simulink model "quadcopter_model"  (R2026a)
settings: Solver=VariableStepAuto  StopTime=60
undefined symbols (not defined in the file): g, Ixx, Iyy, Izz, m
libraries: mpclib x1, uavutilslib x1
settings Model: Creator=Krrrrish  LastModifiedBy=Krrrrish

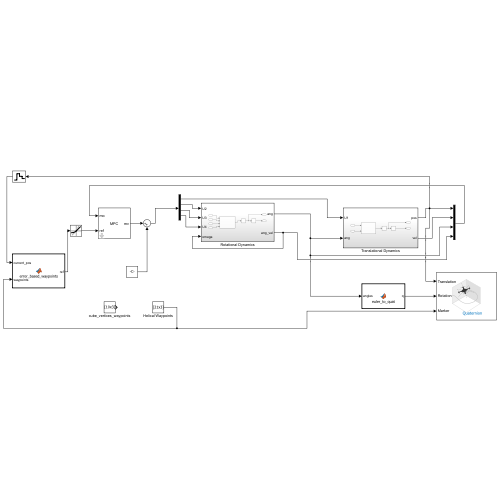
[thumbnail: Simulink's stored preview of the top-level diagram]
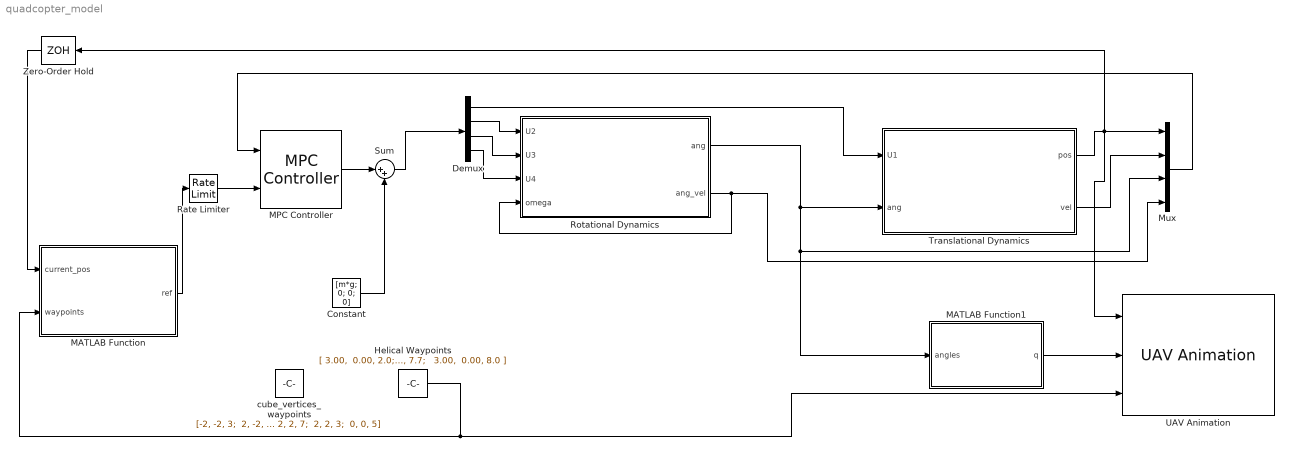
== system quadcopter_model ==
  Constant : Constant  Value=[m*g; 0; 0; 0]
  Demux : Demux
  Helical Waypoints : Constant  Value=|
      | [ 3.00,  0.00, 2.0;
      |   2.43,  1.76, 2.3;
      |   0.93,  2.85, 2.6;
      |  -0.93,  2.85, 2.9;
      |  -2.43,  1.76, 3.2;
      |  -3.00,  0.00, 3.5;
      |  -2.43, -1.76, 3.8;
      |  -0.93, -2.85, 4.1;
      |   0.93, -2.85, 4.4;
      |   2.43, -1.76, 4.7;
      |   3.00,  0.00, 5.0;
      |   2.43,  1.76, 5.3;
      |   0.93,  2.85, 5.6;
      |  -0.93,  2.85, 5.9;
      |  -2.43,  1.76, 6.2;
      |  -3.00,  0.00, 6.5;
      |  -2.43, -1.76, 6.8;
      |  -0.93, -2.85, 7.1;
      |   0.93, -2.85, 7.4;
      |   2.43, -1.76, 7.7;
      |   3.00,  0.00, 8.0 ]
  MATLAB Function : MATLAB Function  TreatAsAtomicUnit=on
  MATLAB Function1 : MATLAB Function  TreatAsAtomicUnit=on
  MPC Controller : mpclib/MPC Controller  SCDEnableBlockLinearizationSpecification=on  mpcobj=mpc_obj  is_multiple=0  enable_value=0  return_u0=off  updateMPCinCallerWorkspace=on  md_inport=off  mv_inport=off  uref_inport=off  return_cost=off  return_mvseq=off  return_qpstatus=off  return_xseq=off  return_state=off  return_ovseq=off  state_inport=off  umin_inport=off  umax_inport=off  ymin_inport=off  ymax_inport=off  cc_inport=off  ywt_inport=off  uwt_inport=off  duwt_inport=off  rhoeps_inport=off  pm_inport=off  MaximumP=10  HorizonChoice=FixedHorizon  n_ts=0.05  n_p=20  n_mv=4  n_md=0  n_ud=0  n_mo=12  n_uo=0  BlockDataType=double  SampleTimeInherited=off  switch_inport=off
  Mux : Mux
  Rate Limiter : RateLimiter  SampleTimeMode=inherited
  Rotational Dynamics : Subsystem
  Sum : Sum  Inputs=|++
  Translational Dynamics : Subsystem
  UAV Animation : uavutilslib/UAV Animation  NumUAV=1  DynamicUAVConfig=off  UAVType=Multirotor  UAVSize=1  UAVColor=[1 0 0]  UAVTrajectoryAlpha=1  AlwaysShowAnimation=on  AxisLimits=[-5 5; -5 5; -10 1]  TrajectoryBufferSize=100000  InertialZDirection=Down  RotationFormat=Quaternion  DrawMarkers=on  SampleTime=-1
  Zero-Order Hold : ZeroOrderHold  SampleTime=-1
  cube_vertices_waypoints : Constant  Value="[-2, -2, 3;  2, -2, 3;  2, 2, 3; -2, 2, 3; -2, 2, 7; -2, -2, 7;  2, -2, 7;  2, 2, 7;  2, 2, 3;  0, 0, 5]"
  wires:
  Rotational Dynamics/2(ang_vel) -> Mux/4, Rotational Dynamics/4(omega)
  Rotational Dynamics/1(ang) -> Translational Dynamics/2(ang), MATLAB Function1/1(angles), Mux/3
  Translational Dynamics/1(pos) -> UAV Animation/1, Zero-Order Hold/1, Mux/1
  Translational Dynamics/2(vel) -> Mux/2
  Constant/1 -> Sum/2
  Sum/1 -> Demux/1
  Demux/4 -> Rotational Dynamics/3(U4)
  Demux/3 -> Rotational Dynamics/2(U3)
  Demux/2 -> Rotational Dynamics/1(U2)
  Demux/1 -> Translational Dynamics/1(U1)
  MPC Controller/1 -> Sum/1
  Mux/1 -> MPC Controller/1
  Zero-Order Hold/1 -> MATLAB Function/1(current_pos)
  MATLAB Function/1(ref) -> Rate Limiter/1
  Rate Limiter/1 -> MPC Controller/2
  MATLAB Function1/1(q) -> UAV Animation/2
  Helical Waypoints/1 -> UAV Animation/3, MATLAB Function/2(waypoints)

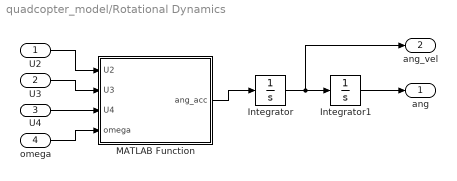
== system quadcopter_model/Rotational Dynamics ==
  U2 : Inport
  U3 : Inport  Port=2
  U4 : Inport  Port=3
  omega : Inport  Port=4
  Integrator : Integrator
  Integrator1 : Integrator
  MATLAB Function : MATLAB Function  TreatAsAtomicUnit=on
  ang : Outport
  ang_vel : Outport  Port=2
  wires:
  MATLAB Function/1(ang_acc) -> Integrator/1
  Integrator/1 -> ang_vel/1, Integrator1/1
  Integrator1/1 -> ang/1
  U2/1 -> MATLAB Function/1(U2)
  U3/1 -> MATLAB Function/2(U3)
  U4/1 -> MATLAB Function/3(U4)
  omega/1 -> MATLAB Function/4(omega)

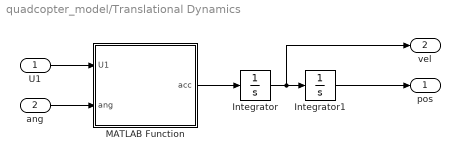
== system quadcopter_model/Translational Dynamics ==
  U1 : Inport
  ang : Inport  Port=2
  Integrator : Integrator
  Integrator1 : Integrator
  MATLAB Function : MATLAB Function  TreatAsAtomicUnit=on
  pos : Outport
  vel : Outport  Port=2
  wires:
  MATLAB Function/1(acc) -> Integrator/1
  Integrator/1 -> vel/1, Integrator1/1
  Integrator1/1 -> pos/1
  U1/1 -> MATLAB Function/1(U1)
  ang/1 -> MATLAB Function/2(ang)

== matlab function quadcopter_model/Rotational Dynamics/MATLAB Function ==
  data: U2 input; U3 input; U4 input; ang_acc output size=[3, 1]; omega input; Ixx parameter; Iyy parameter; Izz parameter
function ang_acc = rot_math(U2, U3, U4, omega, Ixx, Iyy, Izz)
    % 1. Extract current angular velocities (p, q, r) from the omega vector
    p = omega(1); % Roll rate
    q = omega(2); % Pitch rate
    r = omega(3); % Yaw rate
    
    % 2. Apply Euler's Equations of Motion for a rigid body
    % ang_acc = Inverse(Inertia) * (Torques - CrossProduct(omega, Inertia * omega))
    
    p_dot = (U2 + (Iyy - Izz) * q * r) / Ixx;
    q_dot = (U3 + (Izz - Ixx) * p * r) / Iyy;
    r_dot = (U4 + (Ixx - Iyy) * p * q) / Izz;
    
    % Output as a 3x1 column vector
    ang_acc = [p_dot; q_dot; r_dot];
end

== matlab function quadcopter_model/Translational Dynamics/MATLAB Function ==
  data: U1 input; acc output size=[3, 1]; ang input; m parameter; g parameter
function acc = MATLAB_Function(U1, ang, m, g)
acc = zeros(3,1);
% 1. Define Thrust in the Drone's Body Frame
% The motors only push "up" relative to the drone itself (Z-axis)
Thrust_Body = [0; 0; U1];

% 2. Pre-compute sines and cosines for the Rotation Matrix
cphi = cos(ang(1)); sphi = sin(ang(1));
cth  = cos(ang(2)); sth = sin(ang(2));
cpsi = cos(ang(3)); spsi = sin(ang(3));

% 3. Standard Z-Y-X Rotation Matrix (Body Frame to Earth Frame)
R = [ cth*cpsi,  sphi*sth*cpsi - cphi*spsi,  cphi*sth*cpsi + sphi*spsi;
    cth*spsi,  sphi*sth*spsi + cphi*cpsi,  cphi*sth*spsi - sphi*cpsi;
    -sth,       sphi*cth,                   cphi*cth];

% 4. Rotate the body thrust into Earth coordinates
Force_Earth = R * Thrust_Body;

% 5. Calculate Linear Acceleration (F = ma -> a = F/m)
% Note: Gravity only pulls down on the Z-axis
acc_x = Force_Earth(1) / m;
acc_y = Force_Earth(2) / m;
acc_z = (Force_Earth(3) / m) - g;

% Output as a 3x1 column vector
acc = [acc_x; acc_y; acc_z];
end

== matlab function quadcopter_model/MATLAB Function ==
  data: current_pos input; ref output; waypoints input
function ref = error_based_waypoints(current_pos, waypoints)
    % Initialize the 12x1 reference vector
    ref = zeros(12,1);
    
    % Use a 'persistent' variable to remember the waypoint index across time steps
    persistent current_index;
    if isempty(current_index)
        current_index = 1; % Start at the first waypoint
    end
    
    % --- Define the Flight Plan (The Cube) ---
    num_points = size(waypoints, 1);
    
    % --- Calculate Positional Error ---
    % Get the current target coordinates
    target_x = waypoints(current_index, 1);
    target_y = waypoints(current_index, 2);
    target_z = waypoints(current_index, 3);
    
    % Calculate the 3D distance between the drone and the target
    error_distance = sqrt((target_x - current_pos(1))^2 + ...
                          (target_y - current_pos(2))^2 + ...
                          (target_z - current_pos(3))^2);
                          
    % --- The Logic Gate ---
    % If the drone is within 0.3 meters of the target, it has "arrived"
    arrival_threshold = 0.3; 
    
    if (error_distance < arrival_threshold) && (current_index < num_points)
        current_index = current_index + 1; % Move to the next waypoint!
    end
    
    % --- Output the Reference ---
    % Send the current target to the MPC
    ref(1) = waypoints(current_index, 1);
    ref(2) = waypoints(current_index, 2);
    ref(3) = waypoints(current_index, 3);
end

== matlab function quadcopter_model/MATLAB Function1 ==
  data: angles input; q output
function q = euler_to_quat(angles)
    % Pre-allocate the 4x1 output vector
    q = zeros(4,1);
    
    % Extract Euler Angles: [Roll (phi), Pitch (theta), Yaw (psi)]
    phi = angles(1); 
    theta = angles(2); 
    psi = angles(3);
    
    % Calculate half-angles
    c_phi = cos(phi * 0.5);   s_phi = sin(phi * 0.5);
    c_theta = cos(theta * 0.5); s_theta = sin(theta * 0.5);
    c_psi = cos(psi * 0.5);   s_psi = sin(psi * 0.5);
    
    % Convert to standard aerospace Quaternion [w, x, y, z]
    q(1) = c_phi * c_theta * c_psi + s_phi * s_theta * s_psi; % w (scalar)
    q(2) = s_phi * c_theta * c_psi - c_phi * s_theta * s_psi; % x
    q(3) = c_phi * s_theta * c_psi + s_phi * c_theta * s_psi; % y
    q(4) = c_phi * c_theta * s_psi - s_phi * s_theta * c_psi; % z
end
